simulink model "setController2"  (R2020b)
settings: Solver=FixedStepAuto  StartTime=0.0  StopTime=10.0  RelTol=1e-3
values from neighbouring files (symbols this model uses):
  Controller =     [Variables.mat]
  g = 9.81    [Variables.mat]
  Ts = 0.005    [Variables.mat]
  Vehicle =     [Variables.mat]
settings Model: Creator=USER  LastModifiedBy=USER

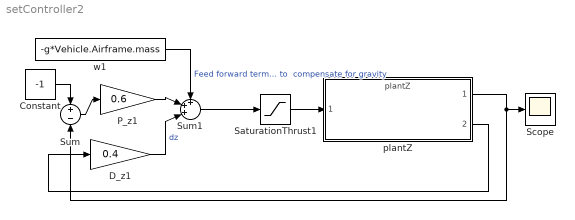
== system setController2 ==
  Constant : Constant  Value=-1  OutDataTypeStr=double
  D_z1 : Gain  Gain=0.4  ParamDataTypeStr=single  OutDataTypeStr=single  SaturateOnIntegerOverflow=on
  P_z1 : Gain  Gain=0.6  ParamDataTypeStr=single  OutDataTypeStr=single  SaturateOnIntegerOverflow=on
  SaturationThrust1 : Saturate  UpperLimit=4*Controller.totalThrustMaxRelative*Controller.motorsThrustPerMotorMax  LowerLimit=-4*Controller.totalThrustMaxRelative*Controller.motorsThrustPerMotorMax  OutDataTypeStr=single
  Scope : Scope
  Sum : Sum  Inputs=+-
  Sum1 : Sum  Inputs=+++|
  plantZ : ModelReference  ModelNameDialog=plantZ  SimulationMode=Normal  ModelReferenceVersion=1.10
  w1 : Constant  Value=-g*Vehicle.Airframe.mass  OutDataTypeStr=single  SampleTime=Ts
  wires:
  Constant/1 -> Sum/1
  Sum/1 -> P_z1/1
  plantZ/1 -> Scope/1, Sum/2
  Sum1/1 -> SaturationThrust1/1
  P_z1/1 -> Sum1/2
  w1/1 -> Sum1/1  "Feed forward term to  compensate for gravity"
  SaturationThrust1/1 -> plantZ/1
  D_z1/1 -> Sum1/3  "dz"
  plantZ/2 -> D_z1/1
